simulink model "modelV1"  (R2024b)
settings: Solver=VariableStepAuto  StartTime=0.0  StopTime=30  RelTol=1e-3
libraries: simulink x1
settings Model: Creator=C27Lucan.Keyser  LastModifiedBy=lucan

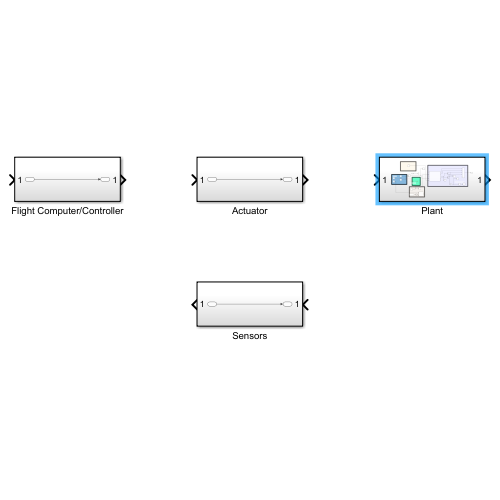
[thumbnail: Simulink's stored preview of the top-level diagram]
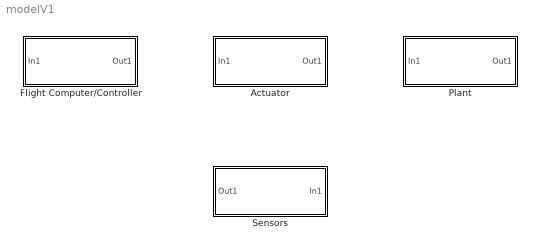
== system modelV1 ==
  Actuator : Subsystem
  Flight Computer/Controller : Subsystem
  Plant : Subsystem
  Sensors : Subsystem

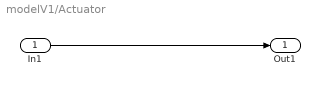
== system modelV1/Actuator ==
  In1 : Inport
  Out1 : Outport
  wires:
  In1/1 -> Out1/1

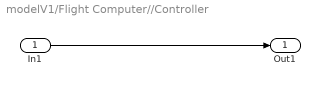
== system modelV1/Flight Computer//Controller ==
  In1 : Inport
  Out1 : Outport
  wires:
  In1/1 -> Out1/1

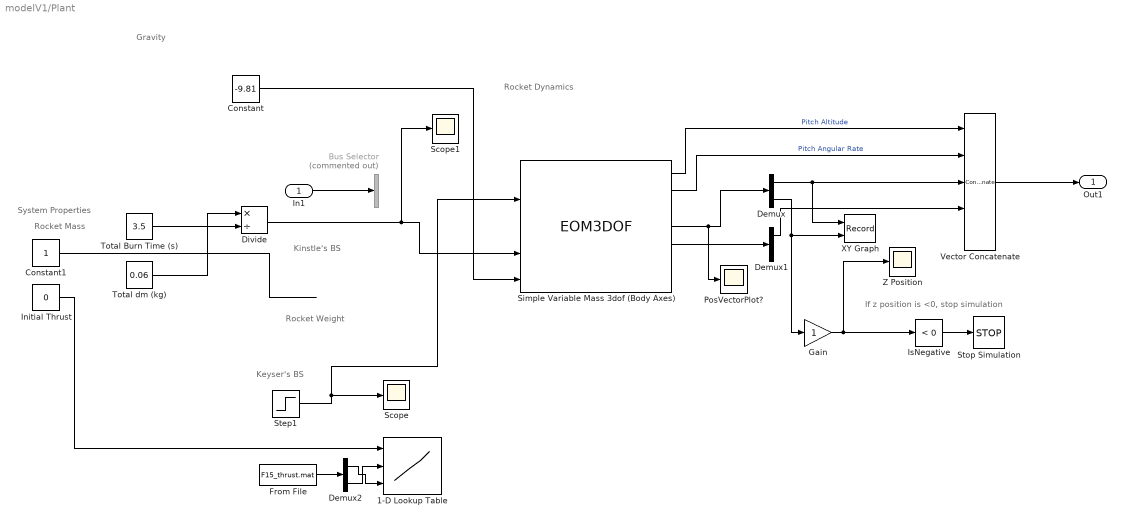
== system modelV1/Plant ==
  note: Kinstle's BS
  note: Rocket Weight
  note: Rocket Mass
  note: System Properties
  note: If z position is <0, stop simulation
  note: Keyser's BS
  note: Gravity
  note: Rocket Dynamics
  In1 : Inport
  1-D Lookup Table : Lookup_n-D  NumberOfTableDimensions=1  BreakpointsForDimension1Source=Input port  BreakpointsForDimension1=[-5:5]  TableSource=Input port  Table=tanh([-5:5])  InternalRulePriority=Speed  RndMeth=Simplest
      settings: InputPortMap=u0,p221,p5
  Bus Selector : BusSelector  Commented=on  OutputSignals=signal1,signal2
  Constant : Constant  Value=-9.81
  Constant1 : Constant
  Demux : Demux  Outputs=2
  Demux1 : Demux  Outputs=2
  Demux2 : Demux  Outputs=2
  Divide : Product  Inputs=*/  OutDataTypeStr=double
  From File : FromFile  FileName=F15_thrust.mat  SampleTime=0
  Gain : Gain
  Initial Thrust : Constant  Value=0
  IsNegative : simulink/Logic and Bit Operations/Compare To Zero  relop=<  OutDataTypeStr=boolean
      settings: LibrarySourceBlock=|
      | simulink/Quick Insert/Logic and Bit
      | Operations/IsNegative
  PosVectorPlot? : Scope
  Scope : Scope
  Scope1 : Scope
  Simple Variable Mass 3dof (Body Axes) : EOM3DOF  mtype=Simple Variable  g_in=External
  Step1 : Step  Time=5  Before=18  After=0  SampleTime=0
  Stop Simulation : Stop
  Total Burn Time (s) : Constant  Value=3.5
  Total dm (kg) : Constant  Value=0.06
  Vector Concatenate : Concatenate  NumInputs=5
  XY Graph : Record  FileSettingsInternal="{\"entries\":[{\"content\":{\"excelSettings\":{\"content\":{},\"type\":\"Streamout.ExcelSettings\"}},\"type\":\"Streamout.FileSettingStorage\",\"uuid\":\"\"}],\"packageUris\":[\"http:\\/\\/schema.mathworks.com\\/mf0\\/streamout_blocks\\/R2020a\"],\"version\":\"1.0\"}"  Layout=[1 1]  SignalsInternal="{\"entries\":[{\"content\":{\"signals\":[{\"content\":{\"blockPath\":[],\"dimensions\":[1],\"domain\":\"\",\"lineColor\":\"#a2142f\",\"plots\":[ 1 ],\"port\":1,\"sid\":[\"\"],\"signalID\":1,\"signalName\":\"Demux:1\"},\"type\":\"RecordBlkView.Signal\",\"uuid\":\"\"},{\"content\":{\"blockPath\":[],\"dimensions\":[1],\"domain\":\"\",\"lineColor\":\"#139fff\",\"plots\":[ 1 ],\"port\":2,\"sid\":[\"\"],\"signalID\":2,\"signalName\":\"Demux:2\"},\"type\":\"RecordBlkView.Signal\",\"uuid\":\"\"}]},\"type\":\"RecordBlkView.InputSignals\",\"uuid\":\"\"}],\"packageUris\":[\"http:\\/\\/schema.mathworks.com\\/mf0\\/streamout_blocks\\/R2020a\"],\"version\":\"1.0\"}"  VisualizationBindings="{\"xyplotplugin\":{\"info\":[{\"series\":[{\"bindingParametersList\":[{\"parameter\":\"X-Axis\",\"signalID\":1,\"signalName\":\"Demux:1\"},{\"parameter\":\"Y-Axis\",\"signalID\":2,\"signalName\":\"Demux:2\"}],\"seriesID\":0}],\"subplotID\":1}]}}"  CompatibilityTag=XY
  Z Position : Scope
  Out1 : Outport
  wires:
  In1/1 -> Bus Selector/1
  Simple Variable Mass 3dof (Body Axes)/1 -> Vector Concatenate/1  "Pitch Altitude"
  Simple Variable Mass 3dof (Body Axes)/2 -> Vector Concatenate/2  "Pitch Angular Rate"
  Simple Variable Mass 3dof (Body Axes)/5 -> Demux1/1
  Simple Variable Mass 3dof (Body Axes)/4 -> PosVectorPlot?/1, Demux/1
  Demux/1 -> XY Graph/1, Vector Concatenate/3
  Demux1/1 -> Vector Concatenate/4
  Vector Concatenate/1 -> Out1/1
  Demux/2 -> XY Graph/2, Gain/1
  Gain/1 -> IsNegative/1, Z Position/1
  IsNegative/1 -> Stop Simulation/1
  Constant1/1 -> ?
  ? -> ?
  Constant/1 -> Simple Variable Mass 3dof (Body Axes)/5
  Initial Thrust/1 -> 1-D Lookup Table/1
  From File/1 -> Demux2/1
  Demux2/1 -> 1-D Lookup Table/3
  Demux2/2 -> 1-D Lookup Table/2
  Step1/1 -> Simple Variable Mass 3dof (Body Axes)/2, Scope/1
  Divide/1 -> Scope1/1, Simple Variable Mass 3dof (Body Axes)/4
  Total dm (kg)/1 -> Divide/1
  Total Burn Time (s)/1 -> Divide/2

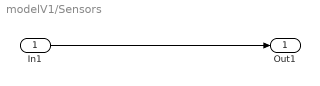
== system modelV1/Sensors ==
  In1 : Inport
  Out1 : Outport
  wires:
  In1/1 -> Out1/1
